simulink model "Subsystem_ProjectModel"  (Simulink 8.0)
settings: Solver=ode45  StartTime=0.0  StopTime=10.0  RelTol=1e-3
values from neighbouring files (symbols this model uses):
  beta_init = 0    [subsystem_bug.m]
  dt_model = 0.2    [subsystem_bug.m]
  l_r = 3    [subsystem_bug.m]
  m_car = 1920    [subsystem_bug.m]
  phi_0 = 0    [subsystem_bug.m]
  x_0 = 0    [subsystem_bug.m]
  x_m = [x_0,y_0,phi_0,0]'    [subsystem_bug.m]
  y_0 = 0    [subsystem_bug.m]
libraries: BLOM_Lib x28
settings Model: Creator=JJK  LastModifiedBy=JJK
settings DataIOCC: SignalLoggingSaveFormat=ModelDataLogs  InspectSignalLogs=on
settings DebuggingCC: MultiTaskDSMMsg=warning  MultiTaskCondExecSysMsg=none
settings RTWCC: IncludeERTFirstTime=on
settings CodeAppCC: CustomSymbolStrType=$N$R$M_T  InternalIdentifier=Shortened

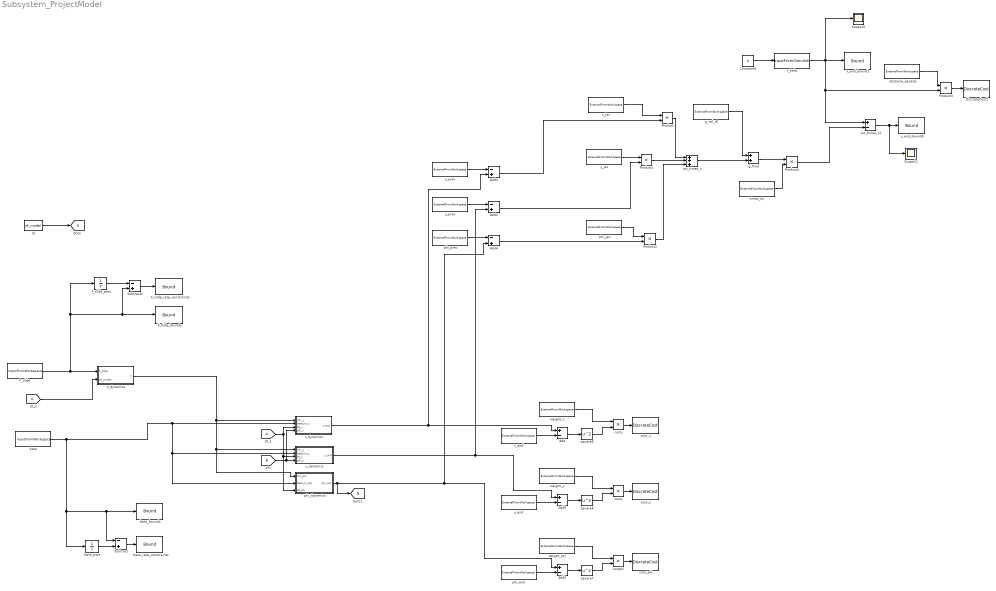
== system Subsystem_ProjectModel ==
  Add : Sum  Inputs=+-
  Add2 : Sum  Inputs=-+
  Add3 : Sum  Inputs=-+
  Add4 : Sum  Inputs=-+
  Add5 : Sum  Inputs=+-
  Add6 : Sum  Inputs=+-
  Constant6 : Constant  Value=0
  DiscreteCost2 : BLOM_Lib/DiscreteCost  initial_step=on  intermediate_step=on  final_step=on
  F_tilde : BLOM_Lib/InputFromWorkspace  simin=F_tilde  interpType=Zero-Order Hold  move_blocking_info=[1 0]
  F_tilde_bounds : BLOM_Lib/Bound  ub=F_tilde_ub  lb=F_tilde_lb  initial_step=on  intermediate_step=on  final_step=on
  F_tilde_past : UnitDelay  SampleTime=-1
  "F_tilde_rate_constraints " : BLOM_Lib/Bound  ub=F_tilde_r_ub  lb=F_tilde_r_lb  initial_step=on  intermediate_step=on  final_step=on
  Product{,1..4} (5 alike) : Product  RndMeth=Zero
  Scope10 : Scope
  Scope11 : Scope
  Subtract : Sum  Inputs=-+
  Subtract2 : Sum  Inputs=-+
  V_dynamics : Subsystem
  beta : BLOM_Lib/InputFromWorkspace  simin=beta  interpType=Zero-Order Hold  move_blocking_info=[1 0]
  beta_bounds : BLOM_Lib/Bound  ub=beta_ub  lb=beta_lb  initial_step=on  intermediate_step=on  final_step=on
  beta_past : UnitDelay  InitialCondition=beta_init  SampleTime=-1
  beta_rate_constraints : BLOM_Lib/Bound  ub=beta_r_ub  lb=beta_r_lb  initial_step=on  intermediate_step=on  final_step=on
  cost_phi : BLOM_Lib/DiscreteCost  initial_step=on  intermediate_step=on  final_step=on
  cost_x : BLOM_Lib/DiscreteCost  initial_step=on  intermediate_step=on  final_step=on
  cost_y : BLOM_Lib/DiscreteCost  initial_step=on  intermediate_step=on  final_step=on
  costphi : Product  RndMeth=Zero
  costx : Product  RndMeth=Zero
  costy : Product  RndMeth=Zero
  dt : Constant  Value=dt_model
  g_final : Sum
  g_val_x0 : BLOM_Lib/ExternalFromWorkspace  simin=g_val_x0  interpType=Zero-Order Hold  move_blocking_info=[1 0]
  jac_times_x : Sum  Inputs=+++
  jac_times_x1 : Sum  Inputs=+-
  obstacle_penalty : BLOM_Lib/ExternalFromWorkspace  simin=obstacle_penalty  interpType=Zero-Order Hold  move_blocking_info=[1 0]
  phi_dynamics : Subsystem
  phi_end : BLOM_Lib/ExternalFromWorkspace  simin=phi_end  interpType=First-Order Hold  move_blocking_info=[1 0]
  phi_jac : BLOM_Lib/ExternalFromWorkspace  simin=phi_jac  interpType=First-Order Hold  move_blocking_info=[1 0]
  phi_prev : BLOM_Lib/ExternalFromWorkspace  simin=phi_prev  interpType=First-Order Hold  move_blocking_info=[1 0]
  square6 : Math  Operator=square  SaturateOnIntegerOverflow=on
  square7 : Math  Operator=square  SaturateOnIntegerOverflow=on
  square8 : Math  Operator=square  SaturateOnIntegerOverflow=on
  t_help : BLOM_Lib/InputFromSimulink  interpType=Zero-Order Hold  move_blocking_info=[1 0]
  times_on : BLOM_Lib/ExternalFromWorkspace  simin=times_on  interpType=Zero-Order Hold  move_blocking_info=[1 0]
  weight_phi : BLOM_Lib/ExternalFromWorkspace  simin=weight_phi  interpType=First-Order Hold  move_blocking_info=[1 0]
  weight_x : BLOM_Lib/ExternalFromWorkspace  simin=weight_x  interpType=First-Order Hold  move_blocking_info=[1 0]
  weight_y : BLOM_Lib/ExternalFromWorkspace  simin=weight_y  interpType=First-Order Hold  move_blocking_info=[1 0]
  x_dynamics : Subsystem
  x_end : BLOM_Lib/ExternalFromWorkspace  simin=x_end  interpType=First-Order Hold  move_blocking_info=[1 0]
  x_end_bound1 : BLOM_Lib/Bound  ub=Inf  lb=0  initial_step=on  intermediate_step=on  final_step=on
  x_end_bound5 : BLOM_Lib/Bound  ub=Inf  lb=0  initial_step=on  intermediate_step=on  final_step=on
  x_jac : BLOM_Lib/ExternalFromWorkspace  simin=x_jac  interpType=First-Order Hold  move_blocking_info=[1 0]
  x_prev : BLOM_Lib/ExternalFromWorkspace  simin=x_prev  interpType=First-Order Hold  move_blocking_info=[1 0]
  y_dynamics : Subsystem
  y_end : BLOM_Lib/ExternalFromWorkspace  simin=y_end  interpType=First-Order Hold  move_blocking_info=[1 0]
  y_jac : BLOM_Lib/ExternalFromWorkspace  simin=y_jac  interpType=First-Order Hold  move_blocking_info=[1 0]
  y_prev : BLOM_Lib/ExternalFromWorkspace  simin=y_prev  interpType=First-Order Hold  move_blocking_info=[1 0]
  tag scope: A=global, B=global
  wires:
  dt/1 -> [A]
  beta_past/1 -> Subtract/2
  Subtract/1 -> beta_rate_constraints/1
  [A] -> x_dynamics/3(dt_x), phi_dynamics/3(dt_phi), y_dynamics/3(dt_y)
  [B] -> x_dynamics/4(phi_x), y_dynamics/4(phi_y)
  x_jac/1 -> Product/1
  y_jac/1 -> Product1/1
  phi_jac/1 -> Product2/1
  Product1/1 -> jac_times_x/2
  Product2/1 -> jac_times_x/3
  Product/1 -> jac_times_x/1
  jac_times_x/1 -> g_final/2
  g_val_x0/1 -> g_final/1
  x_prev/1 -> Add3/1
  y_prev/1 -> Add2/1
  phi_prev/1 -> Add4/1
  Add3/1 -> Product/2
  Add2/1 -> Product1/2
  Add4/1 -> Product2/2
  phi_dynamics/1(phi_out) -> [B], Add5/1, Add4/2
  Product3/1 -> DiscreteCost2/1
  t_help/1 -> Scope10/1, x_end_bound1/1, Product3/2, jac_times_x1/1
  jac_times_x1/1 -> Scope11/1, x_end_bound5/1
  costx/1 -> cost_x/1
  weight_x/1 -> costx/1
  x_end/1 -> Add/2
  Add/1 -> square6/1
  square6/1 -> costx/2
  costphi/1 -> cost_phi/1
  weight_phi/1 -> costphi/1
  phi_end/1 -> Add5/2
  Add5/1 -> square7/1
  square7/1 -> costphi/2
  costy/1 -> cost_y/1
  weight_y/1 -> costy/1
  y_end/1 -> Add6/2
  Add6/1 -> square8/1
  square8/1 -> costy/2
  Constant6/1 -> t_help/1
  x_dynamics/1(x_out) -> Add3/2, Add/1
  y_dynamics/1(y_out) -> Add2/2, Add6/1
  V_dynamics/1(V) -> phi_dynamics/1(Vin_phi), y_dynamics/1(Vin_y), x_dynamics/1(Vin_x)
  [A] -> V_dynamics/2(dt_model)
  beta/1 -> phi_dynamics/2(beta_in_phi), y_dynamics/2(beta_in_y), x_dynamics/2(beta_in_x), Subtract/1, beta_bounds/1, beta_past/1
  F_tilde_past/1 -> Subtract2/1
  Subtract2/1 -> "F_tilde_rate_constraints "/1
  F_tilde/1 -> V_dynamics/1(F_tilde), Subtract2/2, F_tilde_bounds/1, F_tilde_past/1
  obstacle_penalty/1 -> Product3/1
  g_final/1 -> Product4/1
  Product4/1 -> jac_times_x1/2
  times_on/1 -> Product4/2

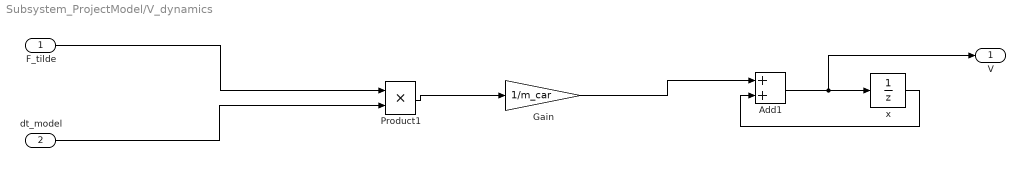
== system Subsystem_ProjectModel/V_dynamics ==
  F_tilde : Inport
  dt_model : Inport  Port=2
  Add1 : Sum
  Gain : Gain  Gain=1/m_car
  Product1 : Product  RndMeth=Zero
  x : UnitDelay  InitialCondition=x_m(4)  SampleTime=-1
  V : Outport
  wires:
  dt_model/1 -> Product1/2
  F_tilde/1 -> Product1/1
  Product1/1 -> Gain/1
  Gain/1 -> Add1/1
  Add1/1 -> V/1, x/1
  x/1 -> Add1/2

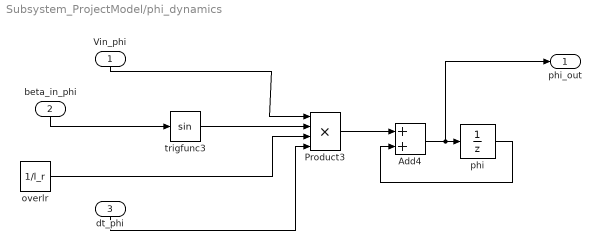
== system Subsystem_ProjectModel/phi_dynamics ==
  Vin_phi : Inport
  beta_in_phi : Inport  Port=2
  dt_phi : Inport  Port=3
  Add4 : Sum
  Product3 : Product  Inputs=4  RndMeth=Zero
  overlr : Constant  Value=1/l_r
  phi : UnitDelay  InitialCondition=phi_0  SampleTime=-1
  trigfunc3 : Trigonometry
  phi_out : Outport
  wires:
  dt_phi/1 -> Product3/4
  trigfunc3/1 -> Product3/2
  overlr/1 -> Product3/3
  Add4/1 -> phi_out/1, phi/1
  Product3/1 -> Add4/1
  phi/1 -> Add4/2
  Vin_phi/1 -> Product3/1
  beta_in_phi/1 -> trigfunc3/1

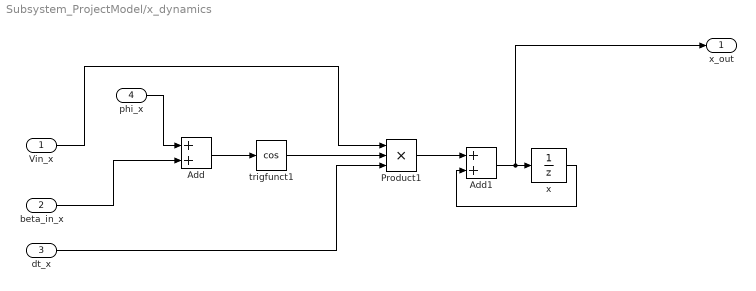
== system Subsystem_ProjectModel/x_dynamics ==
  Vin_x : Inport
  beta_in_x : Inport  Port=2
  dt_x : Inport  Port=3
  phi_x : Inport  Port=4
  Add : Sum
  Add1 : Sum
  Product1 : Product  Inputs=3  RndMeth=Zero
  trigfunct1 : Trigonometry  Operator=cos
  x : UnitDelay  InitialCondition=x_0  SampleTime=-1
  x_out : Outport
  wires:
  beta_in_x/1 -> Add/2
  Add/1 -> trigfunct1/1
  trigfunct1/1 -> Product1/2
  Add1/1 -> x_out/1, x/1
  Product1/1 -> Add1/1
  x/1 -> Add1/2
  dt_x/1 -> Product1/3
  phi_x/1 -> Add/1
  Vin_x/1 -> Product1/1

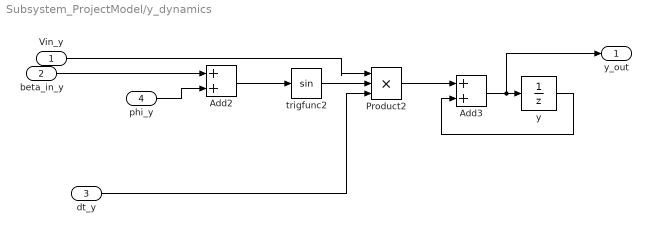
== system Subsystem_ProjectModel/y_dynamics ==
  Vin_y : Inport
  beta_in_y : Inport  Port=2
  dt_y : Inport  Port=3
  phi_y : Inport  Port=4
  Add2 : Sum
  Add3 : Sum
  Product2 : Product  Inputs=3  RndMeth=Zero
  trigfunc2 : Trigonometry
  y : UnitDelay  InitialCondition=y_0  SampleTime=-1
  y_out : Outport
  wires:
  Add2/1 -> trigfunc2/1
  trigfunc2/1 -> Product2/2
  Product2/1 -> Add3/1
  Add3/1 -> y_out/1, y/1
  y/1 -> Add3/2
  dt_y/1 -> Product2/3
  phi_y/1 -> Add2/2
  beta_in_y/1 -> Add2/1
  Vin_y/1 -> Product2/1
